simulink model "main"  (R2023b)
settings: Solver=VariableStepAuto  StartTime=0.0  StopTime=5  RelTol=1e-3
values from neighbouring files (symbols this model uses):
  IMU_sampling_rate = 0.02    [init.m]
  M_Bl = [ALTITUDE YAW -PITCH -ROLL]    [init.m]
  M_Br = [ALTITUDE -YAW -PITCH ROLL]    [init.m]
  M_fl = [ALTITUDE -YAW PITCH -ROLL]    [init.m]
  M_fr = [ALTITUDE YAW PITCH ROLL]    [init.m]
  Ts = 0.02    [init.m]
undefined symbols (not defined in the file or in its folder): dev, DiscIntNeverNeededParam, Main, pwm_output0
libraries: px4Sensorslib x6, slpidlib x4, cstblocks x4, simulink x4, px4lib x3, hdlsllib x2, etargetslib x2, mspfiltlib x1
settings Model: Creator=Jan  LastModifiedBy=Jan

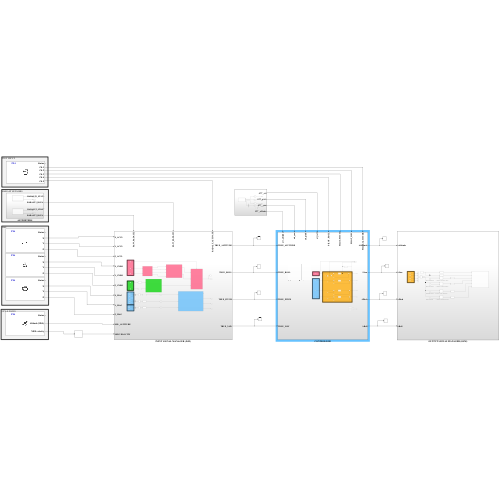
[thumbnail: Simulink's stored preview of the top-level diagram]
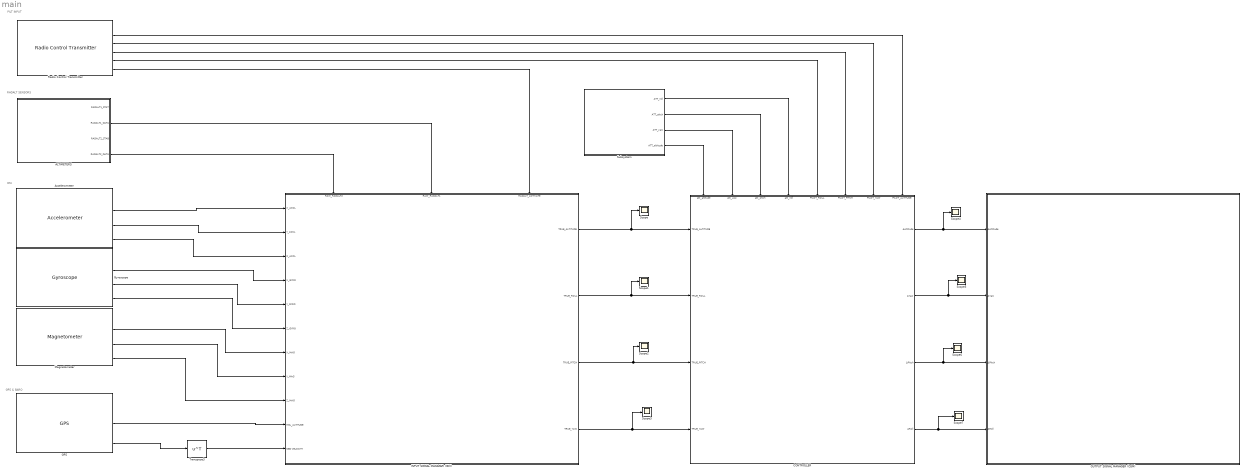
== system main ==
  note: IMU
  note: PILT INPUT
  note: RADALT SENSORS
  note: GPS & BARO
  ALTIMETERS : Subsystem
  Accelerometer : px4Sensorslib/Accelerometer  uorbTimeStamp=off  BlockingMode=off  BlockTimeout=1e-3  sampleTime=1/250
  CONTROLLER : Subsystem
      settings: PortSchema="{\"entries\":[{\"content\":{\"sides\":[{\"content\":{\"connectorIds\":[\"In1\",\"In2\",\"In3\",\"In4\"]},\"type\":\"ConnectorPlacement.EquallySpacedRectSide\",\"uuid\":\"b32f6c27-b4b4-43d4-a12f-bb52559986eb\"},{\"content\":{\"connectorIds\":[\"Out1\",\"Out2\",\"Out3\",\"Out4\"],\"side\":\"RIGHT\"},\"type\":\"ConnectorPlacement.EquallySpacedRectSide\",\"uuid\":\"bab16402-6e46-41ac-967f-b826d0c64ec3\"},{\"content\":{\"connectorIds\":[\"In5\",\"In6\",\"In7\",\"In8\",\"In9\",\"In10\",\"In11\",\"In12\"],\"side\":\"TOP\"},\"type\":\"ConnectorPlacement.EquallySpacedRectSide\",\"uuid\":\"8db3a1c8-77f2-471c-a34f-57b18e4d0f71\"},{\"content\":{\"side\":\"BOTTOM\"},\"type\":\"ConnectorPlacement.EquallySpacedRectSide\",\"uuid\":\"21d3ea43-ab92-4b57-8a2f-eb82c82d00b8\"}]},\"type\":\"ConnectorPlacement.EquallySpacedConnector\",\"uuid\":\"b37a3fa7-6be5-403c-bb68-9dda96af472d\"}],\"packageUris\":[\"http://schema.mathworks.com/mf0/Connector/R2020b\"],\"version\":\"1.0\"}"
  GPS : px4Sensorslib/GPS  lat=off  lon=off  alt=on  velocity=off  course=off  gpsfix=off  numsat=off  timestamp_utc=off  BlockingMode=off  BlockTimeout=1e-3  dop=off  vel_ned=on  alt_ellipsoid=off  jamm_ind=off  timestamp=off  sampleTime=1/250
  Gyroscope : px4Sensorslib/Gyroscope  uorbTimeStamp=off  BlockingMode=off  BlockTimeout=1e-3  sampleTime=1/250
  INPUT SIGNAL MANAGER (ISM) : Subsystem
      settings: PortSchema="{\"entries\":[{\"content\":{\"sides\":[{\"content\":{\"connectorIds\":[\"In1\",\"In2\",\"In3\",\"In4\",\"In5\",\"In6\",\"In7\",\"In8\",\"In9\",\"In10\",\"In11\"]},\"type\":\"ConnectorPlacement.EquallySpacedRectSide\",\"uuid\":\"5b240cc7-ef56-4424-b991-67f01d80d984\"},{\"content\":{\"connectorIds\":[\"Out1\",\"Out2\",\"Out3\",\"Out4\"],\"side\":\"RIGHT\"},\"type\":\"ConnectorPlacement.EquallySpacedRectSide\",\"uuid\":\"4a4e274e-121a-48d3-8cee-a4467ab5abd6\"},{\"content\":{\"connectorIds\":[\"In12\",\"In13\",\"In14\"],\"side\":\"TOP\"},\"type\":\"ConnectorPlacement.EquallySpacedRectSide\",\"uuid\":\"2d4a7b98-56a4-4ac1-89f6-3bfeef007e92\"}]},\"type\":\"ConnectorPlacement.EquallySpacedConnector\",\"uuid\":\"f5ce809e-f10f-4f9c-bc11-40e98aa3c504\"}],\"packageUris\":[\"http://schema.mathworks.com/mf0/Connector/R2020b\"],\"version\":\"1.0\"}"
  Magnetometer : px4Sensorslib/Magnetometer  uorbTimeStamp=off  BlockingMode=off  BlockTimeout=1e-3  sampleTime=1/250
  OUTPUT SIGNAL MANAGER (OSM) : Subsystem
  Radio Control Transmitter : px4Sensorslib/Radio Control Transmitter  channel1=on  channel2=on  channel3=on  channel4=on  channel5=on  channel6=off  channel7=off  channel8=off  channel_count=off  rssi=off  rc_input_source=off  timestamp_last_signal=off  time_stamp=off  sampleTime=1/250  BlockingMode=off  BlockTimeout=5
  Scope{,1..7} (8 alike) : Scope
  Subsystem : Subsystem
  Transpose3 : Math  Operator=transpose
  wires:
  ALTIMETERS/2(RADALT1_DATA) -> INPUT SIGNAL MANAGER (ISM)/13(RAW_RADALT1)
  ALTIMETERS/4(RADALT2_DATA) -> INPUT SIGNAL MANAGER (ISM)/12(RAW_RADALT2)
  Accelerometer/2 -> INPUT SIGNAL MANAGER (ISM)/1(X_ACCL)
  Accelerometer/3 -> INPUT SIGNAL MANAGER (ISM)/2(Y_ACCL)
  Accelerometer/4 -> INPUT SIGNAL MANAGER (ISM)/3(Z_ACCL)
  Gyroscope/2 -> INPUT SIGNAL MANAGER (ISM)/4(X_GYRO)
  Gyroscope/3 -> INPUT SIGNAL MANAGER (ISM)/5(Y_GYRO)
  Gyroscope/4 -> INPUT SIGNAL MANAGER (ISM)/6(Z_GYRO)
  Magnetometer/2 -> INPUT SIGNAL MANAGER (ISM)/7(X_MAG)
  Magnetometer/3 -> INPUT SIGNAL MANAGER (ISM)/8(Y_MAG)
  Magnetometer/4 -> INPUT SIGNAL MANAGER (ISM)/9(Z_MAG)
  GPS/3 -> Transpose3/1
  Transpose3/1 -> INPUT SIGNAL MANAGER (ISM)/11(NED VELOCITY)
  INPUT SIGNAL MANAGER (ISM)/2(TRUE_ROLL) -> Scope1/1, CONTROLLER/2(TRUE_ROLL)
  INPUT SIGNAL MANAGER (ISM)/4(TRUE_YAW) -> Scope3/1, CONTROLLER/4(TRUE_YAW)
  INPUT SIGNAL MANAGER (ISM)/3(TRUE_PITCH) -> Scope2/1, CONTROLLER/3(TRUE_PITCH)
  INPUT SIGNAL MANAGER (ISM)/1(TRUE_ALTITUDE) -> Scope/1, CONTROLLER/1(TRUE_ALTITUDE)
  Radio Control Transmitter/2 -> CONTROLLER/12(PILOT_ALTITUDE)
  Radio Control Transmitter/3 -> CONTROLLER/11(PILOT_YAW)
  Radio Control Transmitter/4 -> CONTROLLER/10(PILOT_PITCH)
  Radio Control Transmitter/5 -> CONTROLLER/9(PILOT_ROLL)
  CONTROLLER/1(ΔAltitude) -> Scope4/1, OUTPUT SIGNAL MANAGER (OSM)/1(ΔAltitude)
  CONTROLLER/2(ΔYaw) -> Scope5/1, OUTPUT SIGNAL MANAGER (OSM)/2(ΔYaw)
  CONTROLLER/3(ΔPitch) -> Scope6/1, OUTPUT SIGNAL MANAGER (OSM)/3(ΔPitch)
  CONTROLLER/4(ΔRoll) -> Scope7/1, OUTPUT SIGNAL MANAGER (OSM)/4(ΔRoll)
  Radio Control Transmitter/6 -> INPUT SIGNAL MANAGER (ISM)/14(RADALT_ACTIVATE)
  Subsystem/4(ATT_altitude) -> CONTROLLER/5(att_altitude)
  Subsystem/3(ATT_yaw) -> CONTROLLER/6(att_yaw)
  Subsystem/2(ATT_pitch) -> CONTROLLER/7(att_pitch)
  Subsystem/1(ATT_roll) -> CONTROLLER/8(att_roll)
  GPS/2 -> INPUT SIGNAL MANAGER (ISM)/10(MSL_ALTITUDE)

== system main/ALTIMETERS ==
  RADALT1 : px4lib/Serial Receive  SCIModule=/dev/ttyS6  DataType=uint8  DataLength=6  OutputStatus=on  SampleTime=1/2400  BlockingMode=off  PartialData=off  Timeout=5
  RADALT2 : px4lib/Serial Receive  SCIModule=/dev/ttyS3  DataType=uint8  DataLength=6  OutputStatus=on  SampleTime=1/2400  BlockingMode=off  PartialData=off  Timeout=5
  RADALT1_STAT : Outport
  RADALT1_DATA : Outport  Port=2
  RADALT2_STAB : Outport  Port=3
  RADALT2_DATA : Outport  Port=4
  wires:
  RADALT2/1 -> RADALT2_DATA/1  "RADALT2"
  RADALT1/1 -> RADALT1_DATA/1  "RADALT1"
  RADALT2/2 -> RADALT2_STAB/1
  RADALT1/2 -> RADALT1_STAT/1

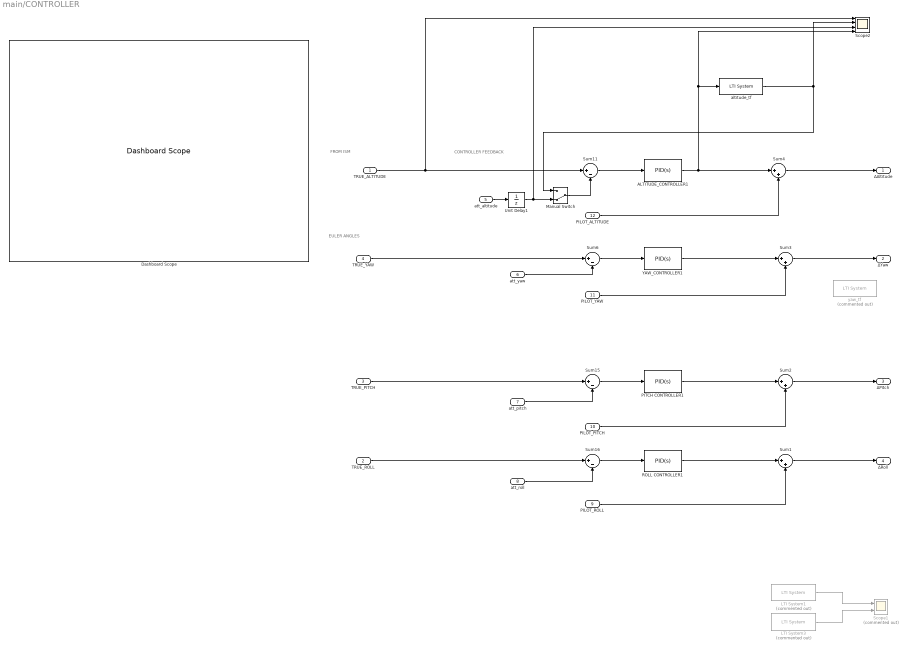
== system main/CONTROLLER ==
  note: EULER ANGLES
  note: FROM ISM
  note: CONTROLLER FEEDBACK
  TRUE_ALTITUDE : Inport
  TRUE_ROLL : Inport  Port=2
  TRUE_PITCH : Inport  Port=3
  TRUE_YAW : Inport  Port=4
  att_altitude : Inport  Port=5
  att_yaw : Inport  Port=6
  att_pitch : Inport  Port=7
  att_roll : Inport  Port=8
  PILOT_ROLL : Inport  Port=9
  PILOT_PITCH : Inport  Port=10
  PILOT_YAW : Inport  Port=11
  PILOT_ALTITUDE : Inport  Port=12
  ALTITUDE_CONTROLLER1 : slpidlib/PID Controller  Controller=PID  Form=Parallel  TimeDomain=Continuous-time  UseExternalTs=off  SampleTime=-1  IntegratorMethod=Forward Euler  FilterMethod=Forward Euler  ControllerParametersSource=internal  P=18932435531.83  I=88617163235.3465  UseKiTs=off  D=988633118.458494  N=575.969167967075  UseFilter=on  TunerSelectOption=Transfer Function Based (PID Tuner App)  InitialConditionSource=internal  InitialConditionForIntegrator=0  InitialConditionForFilter=0  DifferentiatorICPrevScaledInput=0  ExternalReset=none  TrackingMode=off  Kt=1  LimitOutput=off  SatLimitsSource=internal  UpperSaturationLimit=inf  LowerSaturationLimit=-inf  LinearizeAsGain=on  AntiWindupMode=none  Kb=1  LimitIntegrator=off  UpperIntegratorSaturationLimit=inf  LowerIntegratorSaturationLimit=-inf  POutMin=[]  POutMax=[]  IOutMin=[]  IOutMax=[]  DOutMin=[]  DOutMax=[]  NOutMin=[]  NOutMax=[]  SumOutMin=[]  SumOutMax=[]  SaturationOutMin=[]  SaturationOutMax=[]  PParamMin=[]  PParamMax=[]  IParamMin=[]  IParamMax=[]  DParamMin=[]  DParamMax=[]  NParamMin=[]  NParamMax=[]  KbParamMin=[]  KbParamMax=[]  KtParamMin=[]  KtParamMax=[]  KbOutMin=[]  KbOutMax=[]  KtOutMin=[]  KtOutMax=[]  IntegratorOutMin=[]  IntegratorOutMax=[]  FilterOutMin=[]  FilterOutMax=[]  SumI1OutMin=[]  SumI1OutMax=[]  SumI2OutMin=[]  SumI2OutMax=[]  SumI3OutMin=[]  SumI3OutMax=[]  SumI4OutMin=[]  SumI4OutMax=[]  SumDOutMin=[]  SumDOutMax=[]  DifferentiatorOutMin=[]  DifferentiatorOutMax=[]  FilterDiffOutCoefMin=[]  FilterDiffOutCoefMax=[]  ReciprocalOutMin=[]  ReciprocalOutMax=[]  SumDenOutMin=[]  SumDenOutMax=[]  SumNumOutMin=[]  SumNumOutMax=[]  DivideOutMin=[]  DivideOutMax=[]  UdiffTsProdOutMin=[]  UdiffTsProdOutMax=[]  NTsProdOutMin=[]  NTsProdOutMax=[]  UintegralTsProdOutMin=[]  UintegralTsProdOutMax=[]  UngainTsProdOutMin=[]  UngainTsProdOutMax=[]  ClampingZeroOutDataTypeStr=Inherit: Inherit via back propagation  ClampingZeroOutMin=[]  ClampingZeroOutMax=[]  FilterDenConstantOutDataTypeStr=Inherit: Inherit via back propagation  FilterDenConstantOutMin=[]  FilterDenConstantOutMax=[]  PCopyOutDataTypeStr=Inherit: Inherit via back propagation  PCopyOutMin=[]  PCopyOutMax=[]  NCopyOutDataTypeStr=Inherit: Inherit via back propagation  NCopyOutMin=[]  NCopyOutMax=[]  IntegratorContinuousStateAttributes=''  IntegratorStateMustResolveToSignalObject=off  IntegratorRTWStateStorageClass=Auto  FilterContinuousStateAttributes=''  FilterStateMustResolveToSignalObject=off  FilterRTWStateStorageClass=Auto  ParallelPVariant=InternalParameters  IdealPVariant=Disabled  IVariant=InternalParameters  DVariant=InternalParameters  IntegratorVariant=Continuous  SatVariant=Disabled  AWVariant=Passthrough  PCopyVariant=Disabled  TRVariant=Disabled  FdbkBlocksVariant=Forward  IdealPFdbkVariant=Disabled  SatFdbkVariant=Disabled  DerivativeFilterVariant=ContFilter  NVariant=InternalParameters  NCopyVariant=Disabled  FilterICVariant=InternalICsFilter  IntegratorICVariant=InternalICs  ExternalResetVariant=Disabled  TRSumVariant=Passthrough  SumFdbkVariant=Disabled  SumVariant=Sum_PID  TsampFilterVariant=InternalTs  TsampNgainVariant=Passthrough  TsampIntegralVariant=Disabled_SignalSpec  ExternalSaturationOutDataTypeStr=Inherit: Same as second input
  Dashboard Scope : DashboardScope  Ymin=-2  Ymax=10
  LTI System1 : cstblocks/LTI System  Commented=on  sys=pitch_tf  IC=[]  PadeOrder=0
  LTI System3 : cstblocks/LTI System  Commented=on  sys=roll_tf  IC=[]  PadeOrder=0
  Manual Switch : ManualSwitch  CurrentSetting=0
  PITCH CONTROLLER1 : slpidlib/PID Controller  Controller=PID  Form=Parallel  TimeDomain=Continuous-time  UseExternalTs=off  SampleTime=-1  IntegratorMethod=Forward Euler  FilterMethod=Forward Euler  ControllerParametersSource=internal  P=12359690.9371967  I=6312506.2640545  UseKiTs=off  D=5964351.03647163  N=104.897155810233  UseFilter=on  TunerSelectOption=Transfer Function Based (PID Tuner App)  InitialConditionSource=internal  InitialConditionForIntegrator=0  InitialConditionForFilter=0  DifferentiatorICPrevScaledInput=0  ExternalReset=none  TrackingMode=off  Kt=1  LimitOutput=off  SatLimitsSource=internal  UpperSaturationLimit=inf  LowerSaturationLimit=-inf  LinearizeAsGain=on  AntiWindupMode=none  Kb=1  LimitIntegrator=off  UpperIntegratorSaturationLimit=inf  LowerIntegratorSaturationLimit=-inf  POutMin=[]  POutMax=[]  IOutMin=[]  IOutMax=[]  DOutMin=[]  DOutMax=[]  NOutMin=[]  NOutMax=[]  SumOutMin=[]  SumOutMax=[]  SaturationOutMin=[]  SaturationOutMax=[]  PParamMin=[]  PParamMax=[]  IParamMin=[]  IParamMax=[]  DParamMin=[]  DParamMax=[]  NParamMin=[]  NParamMax=[]  KbParamMin=[]  KbParamMax=[]  KtParamMin=[]  KtParamMax=[]  KbOutMin=[]  KbOutMax=[]  KtOutMin=[]  KtOutMax=[]  IntegratorOutMin=[]  IntegratorOutMax=[]  FilterOutMin=[]  FilterOutMax=[]  SumI1OutMin=[]  SumI1OutMax=[]  SumI2OutMin=[]  SumI2OutMax=[]  SumI3OutMin=[]  SumI3OutMax=[]  SumI4OutMin=[]  SumI4OutMax=[]  SumDOutMin=[]  SumDOutMax=[]  DifferentiatorOutMin=[]  DifferentiatorOutMax=[]  FilterDiffOutCoefMin=[]  FilterDiffOutCoefMax=[]  ReciprocalOutMin=[]  ReciprocalOutMax=[]  SumDenOutMin=[]  SumDenOutMax=[]  SumNumOutMin=[]  SumNumOutMax=[]  DivideOutMin=[]  DivideOutMax=[]  UdiffTsProdOutMin=[]  UdiffTsProdOutMax=[]  NTsProdOutMin=[]  NTsProdOutMax=[]  UintegralTsProdOutMin=[]  UintegralTsProdOutMax=[]  UngainTsProdOutMin=[]  UngainTsProdOutMax=[]  ClampingZeroOutDataTypeStr=Inherit: Inherit via back propagation  ClampingZeroOutMin=[]  ClampingZeroOutMax=[]  FilterDenConstantOutDataTypeStr=Inherit: Inherit via back propagation  FilterDenConstantOutMin=[]  FilterDenConstantOutMax=[]  PCopyOutDataTypeStr=Inherit: Inherit via back propagation  PCopyOutMin=[]  PCopyOutMax=[]  NCopyOutDataTypeStr=Inherit: Inherit via back propagation  NCopyOutMin=[]  NCopyOutMax=[]  IntegratorContinuousStateAttributes=''  IntegratorStateMustResolveToSignalObject=off  IntegratorRTWStateStorageClass=Auto  FilterContinuousStateAttributes=''  FilterStateMustResolveToSignalObject=off  FilterRTWStateStorageClass=Auto  ParallelPVariant=InternalParameters  IdealPVariant=Disabled  IVariant=InternalParameters  DVariant=InternalParameters  IntegratorVariant=Continuous  SatVariant=Disabled  AWVariant=Passthrough  PCopyVariant=Disabled  TRVariant=Disabled  FdbkBlocksVariant=Forward  IdealPFdbkVariant=Disabled  SatFdbkVariant=Disabled  DerivativeFilterVariant=ContFilter  NVariant=InternalParameters  NCopyVariant=Disabled  FilterICVariant=InternalICsFilter  IntegratorICVariant=InternalICs  ExternalResetVariant=Disabled  TRSumVariant=Passthrough  SumFdbkVariant=Disabled  SumVariant=Sum_PID  TsampFilterVariant=InternalTs  TsampNgainVariant=Passthrough  TsampIntegralVariant=Disabled_SignalSpec  ExternalSaturationOutDataTypeStr=Inherit: Same as second input
  ROLL CONTROLLER1 : slpidlib/PID Controller  Controller=PID  Form=Parallel  TimeDomain=Continuous-time  UseExternalTs=off  SampleTime=-1  IntegratorMethod=Forward Euler  FilterMethod=Forward Euler  ControllerParametersSource=internal  P=15168306.557733  I=7671855.54074978  UseKiTs=off  D=5885982.08806878  N=104.897155810233  UseFilter=on  TunerSelectOption=Transfer Function Based (PID Tuner App)  InitialConditionSource=internal  InitialConditionForIntegrator=0  InitialConditionForFilter=0  DifferentiatorICPrevScaledInput=0  ExternalReset=none  TrackingMode=off  Kt=1  LimitOutput=off  SatLimitsSource=internal  UpperSaturationLimit=inf  LowerSaturationLimit=-inf  LinearizeAsGain=on  AntiWindupMode=none  Kb=1  LimitIntegrator=off  UpperIntegratorSaturationLimit=inf  LowerIntegratorSaturationLimit=-inf  POutMin=[]  POutMax=[]  IOutMin=[]  IOutMax=[]  DOutMin=[]  DOutMax=[]  NOutMin=[]  NOutMax=[]  SumOutMin=[]  SumOutMax=[]  SaturationOutMin=[]  SaturationOutMax=[]  PParamMin=[]  PParamMax=[]  IParamMin=[]  IParamMax=[]  DParamMin=[]  DParamMax=[]  NParamMin=[]  NParamMax=[]  KbParamMin=[]  KbParamMax=[]  KtParamMin=[]  KtParamMax=[]  KbOutMin=[]  KbOutMax=[]  KtOutMin=[]  KtOutMax=[]  IntegratorOutMin=[]  IntegratorOutMax=[]  FilterOutMin=[]  FilterOutMax=[]  SumI1OutMin=[]  SumI1OutMax=[]  SumI2OutMin=[]  SumI2OutMax=[]  SumI3OutMin=[]  SumI3OutMax=[]  SumI4OutMin=[]  SumI4OutMax=[]  SumDOutMin=[]  SumDOutMax=[]  DifferentiatorOutMin=[]  DifferentiatorOutMax=[]  FilterDiffOutCoefMin=[]  FilterDiffOutCoefMax=[]  ReciprocalOutMin=[]  ReciprocalOutMax=[]  SumDenOutMin=[]  SumDenOutMax=[]  SumNumOutMin=[]  SumNumOutMax=[]  DivideOutMin=[]  DivideOutMax=[]  UdiffTsProdOutMin=[]  UdiffTsProdOutMax=[]  NTsProdOutMin=[]  NTsProdOutMax=[]  UintegralTsProdOutMin=[]  UintegralTsProdOutMax=[]  UngainTsProdOutMin=[]  UngainTsProdOutMax=[]  ClampingZeroOutDataTypeStr=Inherit: Inherit via back propagation  ClampingZeroOutMin=[]  ClampingZeroOutMax=[]  FilterDenConstantOutDataTypeStr=Inherit: Inherit via back propagation  FilterDenConstantOutMin=[]  FilterDenConstantOutMax=[]  PCopyOutDataTypeStr=Inherit: Inherit via back propagation  PCopyOutMin=[]  PCopyOutMax=[]  NCopyOutDataTypeStr=Inherit: Inherit via back propagation  NCopyOutMin=[]  NCopyOutMax=[]  IntegratorContinuousStateAttributes=''  IntegratorStateMustResolveToSignalObject=off  IntegratorRTWStateStorageClass=Auto  FilterContinuousStateAttributes=''  FilterStateMustResolveToSignalObject=off  FilterRTWStateStorageClass=Auto  ParallelPVariant=InternalParameters  IdealPVariant=Disabled  IVariant=InternalParameters  DVariant=InternalParameters  IntegratorVariant=Continuous  SatVariant=Disabled  AWVariant=Passthrough  PCopyVariant=Disabled  TRVariant=Disabled  FdbkBlocksVariant=Forward  IdealPFdbkVariant=Disabled  SatFdbkVariant=Disabled  DerivativeFilterVariant=ContFilter  NVariant=InternalParameters  NCopyVariant=Disabled  FilterICVariant=InternalICsFilter  IntegratorICVariant=InternalICs  ExternalResetVariant=Disabled  TRSumVariant=Passthrough  SumFdbkVariant=Disabled  SumVariant=Sum_PID  TsampFilterVariant=InternalTs  TsampNgainVariant=Passthrough  TsampIntegralVariant=Disabled_SignalSpec  ExternalSaturationOutDataTypeStr=Inherit: Same as second input
  Scope1 : Scope  Commented=on  NumInputPorts=2
  Scope2 : Scope  NumInputPorts=4
  Sum{1..4} (4 alike) : Sum  Inputs=|++
  Sum{6,11,15..16} (4 alike) : Sum  Inputs=|+-
  Unit Delay1 : UnitDelay  SampleTime=-1  HasFrameUpgradeWarning=on
  YAW_CONTROLLER1 : slpidlib/PID Controller  Controller=PID  Form=Parallel  TimeDomain=Continuous-time  UseExternalTs=off  SampleTime=-1  IntegratorMethod=Forward Euler  FilterMethod=Forward Euler  ControllerParametersSource=internal  P=834762470.893906  I=422207783.259263  UseKiTs=off  D=323925214.246719  N=104.897155810233  UseFilter=on  TunerSelectOption=Transfer Function Based (PID Tuner App)  InitialConditionSource=internal  InitialConditionForIntegrator=0  InitialConditionForFilter=0  DifferentiatorICPrevScaledInput=0  ExternalReset=none  TrackingMode=off  Kt=1  LimitOutput=off  SatLimitsSource=internal  UpperSaturationLimit=inf  LowerSaturationLimit=-inf  LinearizeAsGain=on  AntiWindupMode=none  Kb=1  LimitIntegrator=off  UpperIntegratorSaturationLimit=inf  LowerIntegratorSaturationLimit=-inf  POutMin=[]  POutMax=[]  IOutMin=[]  IOutMax=[]  DOutMin=[]  DOutMax=[]  NOutMin=[]  NOutMax=[]  SumOutMin=[]  SumOutMax=[]  SaturationOutMin=[]  SaturationOutMax=[]  PParamMin=[]  PParamMax=[]  IParamMin=[]  IParamMax=[]  DParamMin=[]  DParamMax=[]  NParamMin=[]  NParamMax=[]  KbParamMin=[]  KbParamMax=[]  KtParamMin=[]  KtParamMax=[]  KbOutMin=[]  KbOutMax=[]  KtOutMin=[]  KtOutMax=[]  IntegratorOutMin=[]  IntegratorOutMax=[]  FilterOutMin=[]  FilterOutMax=[]  SumI1OutMin=[]  SumI1OutMax=[]  SumI2OutMin=[]  SumI2OutMax=[]  SumI3OutMin=[]  SumI3OutMax=[]  SumI4OutMin=[]  SumI4OutMax=[]  SumDOutMin=[]  SumDOutMax=[]  DifferentiatorOutMin=[]  DifferentiatorOutMax=[]  FilterDiffOutCoefMin=[]  FilterDiffOutCoefMax=[]  ReciprocalOutMin=[]  ReciprocalOutMax=[]  SumDenOutMin=[]  SumDenOutMax=[]  SumNumOutMin=[]  SumNumOutMax=[]  DivideOutMin=[]  DivideOutMax=[]  UdiffTsProdOutMin=[]  UdiffTsProdOutMax=[]  NTsProdOutMin=[]  NTsProdOutMax=[]  UintegralTsProdOutMin=[]  UintegralTsProdOutMax=[]  UngainTsProdOutMin=[]  UngainTsProdOutMax=[]  ClampingZeroOutDataTypeStr=Inherit: Inherit via back propagation  ClampingZeroOutMin=[]  ClampingZeroOutMax=[]  FilterDenConstantOutDataTypeStr=Inherit: Inherit via back propagation  FilterDenConstantOutMin=[]  FilterDenConstantOutMax=[]  PCopyOutDataTypeStr=Inherit: Inherit via back propagation  PCopyOutMin=[]  PCopyOutMax=[]  NCopyOutDataTypeStr=Inherit: Inherit via back propagation  NCopyOutMin=[]  NCopyOutMax=[]  IntegratorContinuousStateAttributes=''  IntegratorStateMustResolveToSignalObject=off  IntegratorRTWStateStorageClass=Auto  FilterContinuousStateAttributes=''  FilterStateMustResolveToSignalObject=off  FilterRTWStateStorageClass=Auto  ParallelPVariant=InternalParameters  IdealPVariant=Disabled  IVariant=InternalParameters  DVariant=InternalParameters  IntegratorVariant=Continuous  SatVariant=Disabled  AWVariant=Passthrough  PCopyVariant=Disabled  TRVariant=Disabled  FdbkBlocksVariant=Forward  IdealPFdbkVariant=Disabled  SatFdbkVariant=Disabled  DerivativeFilterVariant=ContFilter  NVariant=InternalParameters  NCopyVariant=Disabled  FilterICVariant=InternalICsFilter  IntegratorICVariant=InternalICs  ExternalResetVariant=Disabled  TRSumVariant=Passthrough  SumFdbkVariant=Disabled  SumVariant=Sum_PID  TsampFilterVariant=InternalTs  TsampNgainVariant=Passthrough  TsampIntegralVariant=Disabled_SignalSpec  ExternalSaturationOutDataTypeStr=Inherit: Same as second input
  altitude_tf : cstblocks/LTI System  sys=altitude_tf  IC=[]  PadeOrder=0
  yaw_tf : cstblocks/LTI System  Commented=on  sys=yaw_tf  IC=[]  PadeOrder=0
  ΔAltitude : Outport
  ΔYaw : Outport  Port=2
  ΔPitch : Outport  Port=3
  ΔRoll : Outport  Port=4
  wires:
  YAW_CONTROLLER1/1 -> Sum3/1
  Sum4/1 -> ΔAltitude/1
  ROLL CONTROLLER1/1 -> Sum1/1
  PILOT_ALTITUDE/1 -> Sum4/2
  PILOT_YAW/1 -> Sum3/2
  Sum16/1 -> ROLL CONTROLLER1/1
  Sum1/1 -> ΔRoll/1
  PILOT_ROLL/1 -> Sum1/2
  PITCH CONTROLLER1/1 -> Sum2/1
  Sum15/1 -> PITCH CONTROLLER1/1
  ALTITUDE_CONTROLLER1/1 -> Scope2/4, altitude_tf/1, Sum4/1
  Sum2/1 -> ΔPitch/1
  PILOT_PITCH/1 -> Sum2/2
  Sum11/1 -> ALTITUDE_CONTROLLER1/1
  Sum6/1 -> YAW_CONTROLLER1/1
  TRUE_ROLL/1 -> Sum16/1
  TRUE_PITCH/1 -> Sum15/1
  TRUE_YAW/1 -> Sum6/1
  TRUE_ALTITUDE/1 -> Scope2/1, Sum11/1
  att_yaw/1 -> Sum6/2
  att_pitch/1 -> Sum15/2
  att_roll/1 -> Sum16/2
  Sum3/1 -> ΔYaw/1
  LTI System1/1 -> Scope1/1
  LTI System3/1 -> Scope1/2
  Manual Switch/1 -> Sum11/2
  altitude_tf/1 -> Manual Switch/1, Scope2/2
  Unit Delay1/1 -> Scope2/3, Manual Switch/2
  att_altitude/1 -> Unit Delay1/1

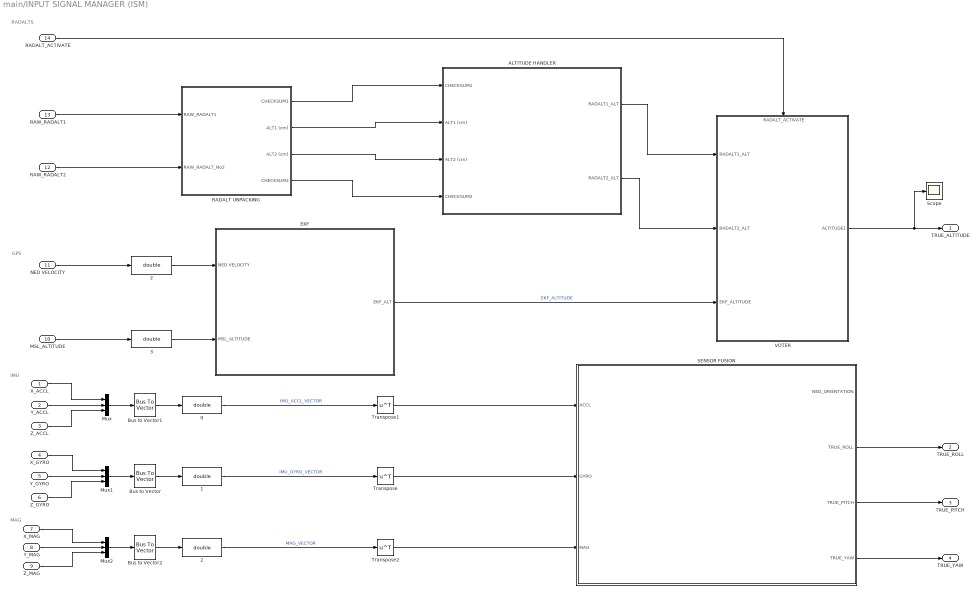
== system main/INPUT SIGNAL MANAGER (ISM) ==
  note: GPS
  note: RADALTS
  note: IMU
  note: MAG
  X_ACCL : Inport
  Y_ACCL : Inport  Port=2
  Z_ACCL : Inport  Port=3
  X_GYRO : Inport  Port=4
  Y_GYRO : Inport  Port=5
  Z_GYRO : Inport  Port=6
  X_MAG : Inport  Port=7
  Y_MAG : Inport  Port=8
  Z_MAG : Inport  Port=9
  MSL_ALTITUDE : Inport  Port=10
  NED VELOCITY : Inport  Port=11
  RAW_RADALT2 : Inport  Port=12
  RAW_RADALT1 : Inport  Port=13
  RADALT_ACTIVATE : Inport  Port=14
  " 2" : DataTypeConversion  OutDataTypeStr=double  SaturateOnIntegerOverflow=off  RndMeth=Floor
  "0 " : DataTypeConversion  OutDataTypeStr=double  SaturateOnIntegerOverflow=off  RndMeth=Floor
  1 : DataTypeConversion  OutDataTypeStr=double  SaturateOnIntegerOverflow=off  RndMeth=Floor
  2 : DataTypeConversion  OutDataTypeStr=double  SaturateOnIntegerOverflow=off  RndMeth=Floor
  3 : DataTypeConversion  OutDataTypeStr=double  SaturateOnIntegerOverflow=off  RndMeth=Floor
  ALTITUDE HANDLER : Subsystem
  Bus to Vector : BusToVector
  Bus to Vector1 : BusToVector
  Bus to Vector2 : BusToVector
  EKF : Subsystem
  Mux : Mux  Inputs=3
  Mux1 : Mux  Inputs=3
  Mux2 : Mux  Inputs=3
  RADALT UNPACKING : Subsystem
  SENSOR FUSION : Subsystem
  Scope : Scope
  Transpose : Math  Operator=transpose
  Transpose1 : Math  Operator=transpose
  Transpose2 : Math  Operator=transpose
  VOTER : Subsystem
      settings: PortSchema="{\"entries\":[{\"content\":{\"sides\":[{\"content\":{\"connectorIds\":[\"In1\",\"In2\",\"In3\"]},\"type\":\"ConnectorPlacement.EquallySpacedRectSide\",\"uuid\":\"dc1c39ce-0403-459b-94e1-ddedc0ea1ee4\"},{\"content\":{\"connectorIds\":[\"Out1\"],\"side\":\"RIGHT\"},\"type\":\"ConnectorPlacement.EquallySpacedRectSide\",\"uuid\":\"853442a8-64b8-4778-9114-161db545e8e2\"},{\"content\":{\"connectorIds\":[\"In4\"],\"side\":\"TOP\"},\"type\":\"ConnectorPlacement.EquallySpacedRectSide\",\"uuid\":\"2ebd7c90-ed78-4be6-83fb-fb9bd20822eb\"}]},\"type\":\"ConnectorPlacement.EquallySpacedConnector\",\"uuid\":\"d02cc3c8-2437-46b2-8909-af6c76dce3d6\"}],\"packageUris\":[\"http://schema.mathworks.com/mf0/Connector/R2020b\"],\"version\":\"1.0\"}"
  TRUE_ALTITUDE : Outport
  TRUE_ROLL : Outport  Port=2
  TRUE_PITCH : Outport  Port=3
  TRUE_YAW : Outport  Port=4
  wires:
  RAW_RADALT1/1 -> RADALT UNPACKING/1(RAW_RADALT1)
  RAW_RADALT2/1 -> RADALT UNPACKING/2(RAW_RADALT_No2)
  RADALT UNPACKING/2(ALT1 (cm)) -> ALTITUDE HANDLER/2(ALT1 (cm))
  RADALT UNPACKING/3(ALT2 (cm)) -> ALTITUDE HANDLER/3(ALT2 (cm))
  RADALT UNPACKING/1(CHECKSUM1) -> ALTITUDE HANDLER/1(CHECKSUM1)
  RADALT UNPACKING/4(CHECKSUM2) -> ALTITUDE HANDLER/4(CHECKSUM2)
  X_ACCL/1 -> Mux/1
  Y_ACCL/1 -> Mux/2
  Z_ACCL/1 -> Mux/3
  X_GYRO/1 -> Mux1/1
  Y_GYRO/1 -> Mux1/2
  Z_GYRO/1 -> Mux1/3
  Mux/1 -> Bus to Vector1/1
  Mux1/1 -> Bus to Vector/1
  Mux2/1 -> Bus to Vector2/1
  Y_MAG/1 -> Mux2/2
  Z_MAG/1 -> Mux2/3
  X_MAG/1 -> Mux2/1
  " 2"/1 -> Transpose2/1  "MAG_VECTOR"
  "0 "/1 -> Transpose1/1  "IMU_ACCL_VECTOR"
  1/1 -> Transpose/1  "IMU_GYRO_VECTOR"
  NED VELOCITY/1 -> 2/1
  Transpose/1 -> SENSOR FUSION/2(GYRO)
  Transpose1/1 -> SENSOR FUSION/1(ACCL)
  Transpose2/1 -> SENSOR FUSION/3(MAG)
  SENSOR FUSION/3(TRUE_PITCH) -> TRUE_PITCH/1
  SENSOR FUSION/2(TRUE_ROLL) -> TRUE_ROLL/1
  SENSOR FUSION/4(TRUE_YAW) -> TRUE_YAW/1
  ALTITUDE HANDLER/1(RADALT1_ALT) -> VOTER/1(RADALT1_ALT)
  ALTITUDE HANDLER/2(RADALT2_ALT) -> VOTER/2(RADALT2_ALT)
  VOTER/1(ALTITUDE1) -> Scope/1, TRUE_ALTITUDE/1
  Bus to Vector2/1 -> " 2"/1
  Bus to Vector/1 -> 1/1
  Bus to Vector1/1 -> "0 "/1
  MSL_ALTITUDE/1 -> 3/1
  RADALT_ACTIVATE/1 -> VOTER/4(RADALT_ACTIVATE)
  EKF/1(EKF_ALT) -> VOTER/3(EKF_ALTITUDE)  "EKF_ALTITUDE"
  2/1 -> EKF/1(NED VELOCITY)
  3/1 -> EKF/2(MSL_ALTITUDE)

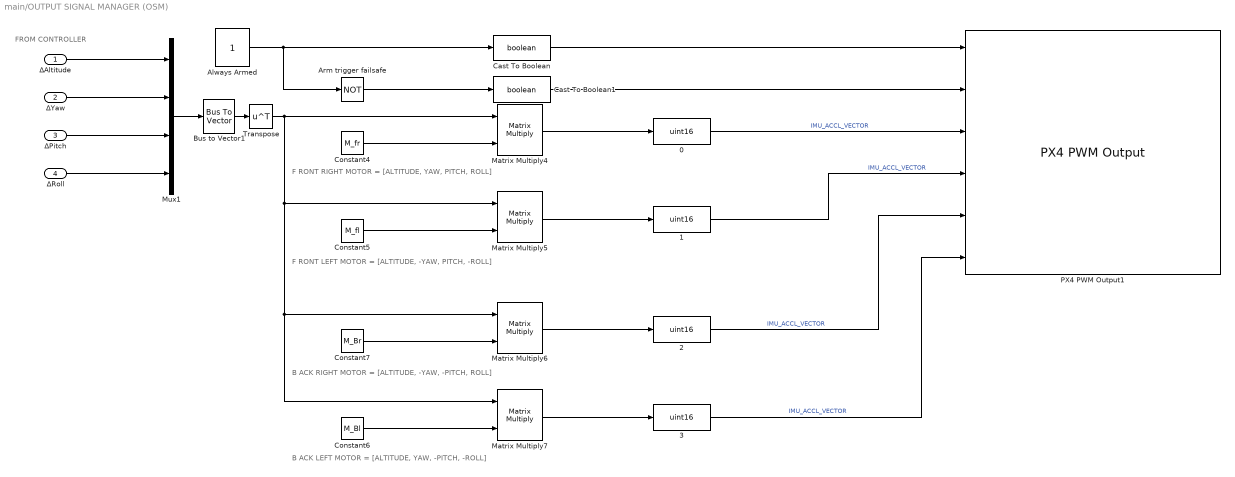
== system main/OUTPUT SIGNAL MANAGER (OSM) ==
  note: FROM CONTROLLER
  note: B ACK LEFT MOTOR = [ALTITUDE, YAW, -PITCH, -ROLL]
  note: F RONT LEFT MOTOR = [ALTITUDE, -YAW, PITCH, -ROLL]
  note: B ACK RIGHT MOTOR = [ALTITUDE, -YAW, -PITCH, ROLL]
  note: F RONT RIGHT MOTOR = [ALTITUDE, YAW, PITCH, ROLL]
  ΔAltitude : Inport
  ΔYaw : Inport  Port=2
  ΔPitch : Inport  Port=3
  ΔRoll : Inport  Port=4
  {0..3} (4 alike) : DataTypeConversion  OutDataTypeStr=uint16  SaturateOnIntegerOverflow=off  RndMeth=Floor
  Always Armed : Constant
  Arm trigger failsafe : Logic  Operator=NOT  IconShape=distinctive  AllPortsSameDT=off  OutDataTypeStr=boolean
  Bus to Vector1 : BusToVector
  Cast To Boolean : DataTypeConversion  OutDataTypeStr=boolean  SaturateOnIntegerOverflow=off  RndMeth=Floor
  Cast To Boolean1 : DataTypeConversion  OutDataTypeStr=boolean  SaturateOnIntegerOverflow=off  RndMeth=Floor
  Constant4 : Constant  Value=M_fr
  Constant5 : Constant  Value=M_fl
  Constant6 : Constant  Value=M_Bl
  Constant7 : Constant  Value=M_Br
  Matrix Multiply{4..7} (4 alike) : Product  Multiplication=Matrix(*)
  Mux1 : Mux
  PX4 PWM Output1 : px4lib/PX4 PWM Output  pwmDevice=Main (/dev/pwm_output0)  pwmChannel1_=on  pwmChannel2_=on  pwmChannel3_=on  pwmChannel4_=on  pwmChannel5_=off  pwmChannel6_=off  pwmChannel7_=off  pwmChannel8_=off  forceTerminateFailsafe=off  outputErrorStatus=off
  Transpose : Math  Operator=transpose
  wires:
  Constant6/1 -> Matrix Multiply7/2
  ΔRoll/1 -> Mux1/4
  ΔAltitude/1 -> Mux1/1
  ΔYaw/1 -> Mux1/2
  ΔPitch/1 -> Mux1/3
  Mux1/1 -> Bus to Vector1/1
  Bus to Vector1/1 -> Transpose/1
  Constant4/1 -> Matrix Multiply4/2
  Constant7/1 -> Matrix Multiply6/2
  Always Armed/1 -> Cast To Boolean/1, Arm trigger failsafe/1
  Constant5/1 -> Matrix Multiply5/2
  Arm trigger failsafe/1 -> Cast To Boolean1/1
  Matrix Multiply5/1 -> 1/1
  1/1 -> PX4 PWM Output1/4  "IMU_ACCL_VECTOR"
  Matrix Multiply4/1 -> 0/1
  0/1 -> PX4 PWM Output1/3  "IMU_ACCL_VECTOR"
  Matrix Multiply6/1 -> 2/1
  2/1 -> PX4 PWM Output1/5  "IMU_ACCL_VECTOR"
  Matrix Multiply7/1 -> 3/1
  3/1 -> PX4 PWM Output1/6  "IMU_ACCL_VECTOR"
  Transpose/1 -> Matrix Multiply5/1, Matrix Multiply7/1, Matrix Multiply6/1, Matrix Multiply4/1
  Cast To Boolean/1 -> PX4 PWM Output1/1
  Cast To Boolean1/1 -> PX4 PWM Output1/2

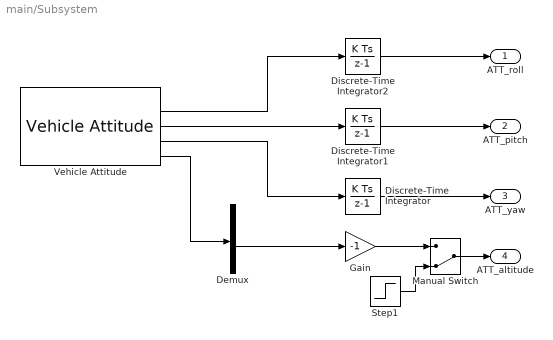
== system main/Subsystem ==
  Demux : Demux
  Discrete-Time Integrator : DiscreteIntegrator  SampleTime=-1  ICPrevOutput=DiscIntNeverNeededParam  ICPrevScaledInput=DiscIntNeverNeededParam
  Discrete-Time Integrator1 : DiscreteIntegrator  SampleTime=-1  ICPrevOutput=DiscIntNeverNeededParam  ICPrevScaledInput=DiscIntNeverNeededParam
  Discrete-Time Integrator2 : DiscreteIntegrator  SampleTime=-1  ICPrevOutput=DiscIntNeverNeededParam  ICPrevScaledInput=DiscIntNeverNeededParam
  Gain : Gain  Gain=-1
  Manual Switch : ManualSwitch  CurrentSetting=0
  Step1 : Step  Time=10  Before=5  After=5  SampleTime=10
  Vehicle Attitude : px4Sensorslib/Vehicle Attitude  rollRate=on  pitchRate=on  yawRate=on  quaternion=on  uorbTimeStamp=off  BlockingMode=off  BlockTimeout=0.001  sampleTime=1/250
  ATT_roll : Outport
  ATT_pitch : Outport  Port=2
  ATT_yaw : Outport  Port=3
  ATT_altitude : Outport  Port=4
  wires:
  Vehicle Attitude/5 -> Demux/1
  Demux/3 -> Gain/1
  Vehicle Attitude/4 -> Discrete-Time Integrator/1
  Vehicle Attitude/3 -> Discrete-Time Integrator1/1
  Vehicle Attitude/2 -> Discrete-Time Integrator2/1
  Discrete-Time Integrator2/1 -> ATT_roll/1
  Discrete-Time Integrator1/1 -> ATT_pitch/1
  Discrete-Time Integrator/1 -> ATT_yaw/1
  Gain/1 -> Manual Switch/1
  Step1/1 -> Manual Switch/2
  Manual Switch/1 -> ATT_altitude/1

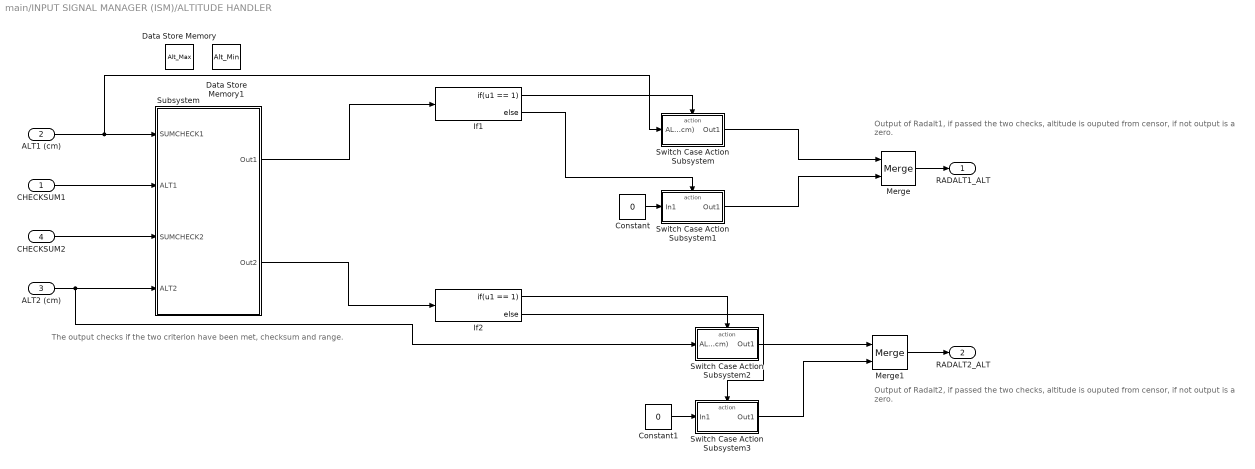
== system main/INPUT SIGNAL MANAGER (ISM)/ALTITUDE HANDLER ==
  note: The output checks if the two criterion have been met, checksum and range.
  note: Output of Radalt2, if passed the two checks, altitude is ouputed from censor, if not output is a zero.
  note: Output of Radalt1, if passed the two checks, altitude is ouputed from censor, if not output is a zero.
  CHECKSUM1 : Inport
  ALT1 (cm) : Inport  Port=2
  ALT2 (cm) : Inport  Port=3
  CHECKSUM2 : Inport  Port=4
  Constant : Constant  Value=0
  Constant1 : Constant  Value=0
  Data Store Memory : DataStoreMemory  DataStoreName=Alt_Max  WriteAfterWriteMsg=warning  ShowAdditionalParam=off
  Data Store Memory1 : DataStoreMemory  DataStoreName=Alt_Min  WriteAfterWriteMsg=warning  ShowAdditionalParam=off
  If1 : If  IfExpression=u1 == 1
  If2 : If  IfExpression=u1 == 1
  Merge : Merge
  Merge1 : Merge
  Subsystem : Subsystem
  Switch Case Action Subsystem : Subsystem  TreatAsAtomicUnit=on
  Switch Case Action Subsystem1 : Subsystem  TreatAsAtomicUnit=on
  Switch Case Action Subsystem2 : Subsystem  TreatAsAtomicUnit=on
  Switch Case Action Subsystem3 : Subsystem  TreatAsAtomicUnit=on
  RADALT1_ALT : Outport
  RADALT2_ALT : Outport  Port=2
  wires:
  Switch Case Action Subsystem3/1(Out1) -> Merge1/2
  Merge/1 -> RADALT1_ALT/1
  Merge1/1 -> RADALT2_ALT/1
  CHECKSUM1/1 -> Subsystem/2(ALT1)
  Switch Case Action Subsystem1/1(Out1) -> Merge/2
  If2/2 -> Switch Case Action Subsystem3/Action
  CHECKSUM2/1 -> Subsystem/3(SUMCHECK2)
  ALT2 (cm)/1 -> Switch Case Action Subsystem2/1(ALT2 (cm)), Subsystem/4(ALT2)
  If1/1 -> Switch Case Action Subsystem/Action
  Switch Case Action Subsystem2/1(Out1) -> Merge1/1
  If1/2 -> Switch Case Action Subsystem1/Action
  Subsystem/1(Out1) -> If1/1
  If2/1 -> Switch Case Action Subsystem2/Action
  Constant/1 -> Switch Case Action Subsystem1/1(In1)
  ALT1 (cm)/1 -> Switch Case Action Subsystem/1(ALT1 (cm)), Subsystem/1(SUMCHECK1)
  Constant1/1 -> Switch Case Action Subsystem3/1(In1)
  Switch Case Action Subsystem/1(Out1) -> Merge/1
  Subsystem/2(Out2) -> If2/1

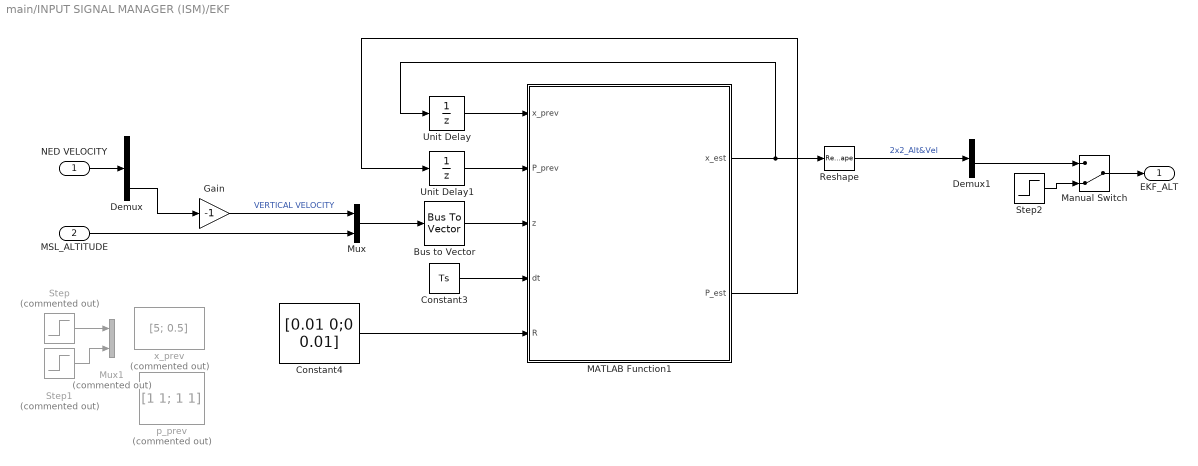
== system main/INPUT SIGNAL MANAGER (ISM)/EKF ==
  NED VELOCITY : Inport
  MSL_ALTITUDE : Inport  Port=2
  Bus to Vector : BusToVector
  Constant3 : Constant  Value=Ts
  Constant4 : Constant  Value=[0.01 0;0 0.01]
  Demux : Demux  Outputs=3
  Demux1 : Demux
  Gain : Gain  Gain=-1
  MATLAB Function1 : MATLAB Function  TreatAsAtomicUnit=on
  Manual Switch : ManualSwitch  CurrentSetting=0
  Mux : Mux  Inputs=2
  Mux1 : Mux  Commented=on  Inputs=2
  Reshape : Reshape
  Step : Step  Commented=on  Time=5  Before=5  After=5  SampleTime=0.02
  Step1 : Step  Commented=on  Time=5  Before=0.5  After=0.5  SampleTime=0.02
  Step2 : Step  Time=10  Before=5  After=5  SampleTime=1
  Unit Delay : UnitDelay  SampleTime=-1  HasFrameUpgradeWarning=on
  Unit Delay1 : UnitDelay  SampleTime=-1  HasFrameUpgradeWarning=on
  p_prev : Constant  Commented=on  Value=[1 1; 1 1]
  x_prev : Constant  Commented=on  Value=[5; 0.5]
  EKF_ALT : Outport
  wires:
  MSL_ALTITUDE/1 -> Mux/2
  Mux/1 -> Bus to Vector/1
  MATLAB Function1/2(P_est) -> Unit Delay1/1
  Constant4/1 -> MATLAB Function1/5(R)
  MATLAB Function1/1(x_est) -> Reshape/1, Unit Delay/1
  Unit Delay/1 -> MATLAB Function1/1(x_prev)
  Bus to Vector/1 -> MATLAB Function1/3(z)
  Constant3/1 -> MATLAB Function1/4(dt)
  Unit Delay1/1 -> MATLAB Function1/2(P_prev)
  Step1/1 -> Mux1/2
  Step/1 -> Mux1/1
  NED VELOCITY/1 -> Demux/1
  Demux/3 -> Gain/1
  Gain/1 -> Mux/1  "VERTICAL VELOCITY"
  Reshape/1 -> Demux1/1  "2x2_Alt&Vel"
  Step2/1 -> Manual Switch/2
  Demux1/3 -> Manual Switch/1
  Manual Switch/1 -> EKF_ALT/1

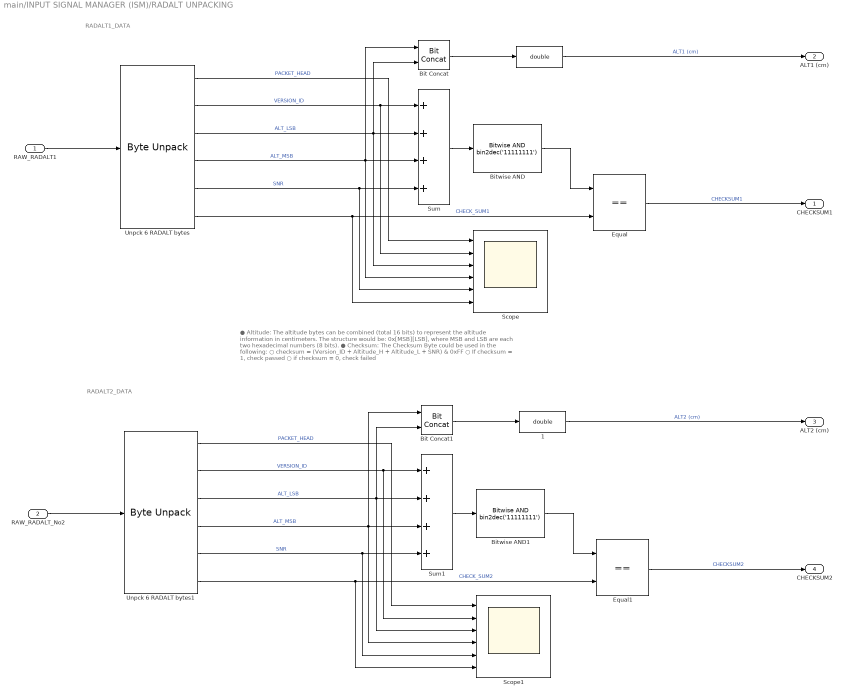
== system main/INPUT SIGNAL MANAGER (ISM)/RADALT UNPACKING ==
  note: RADALT2_DATA
  note: RADALT1_DATA
  note: ● Altitude: The altitude bytes can be combined (total 16 bits) to represent the altitude information in centimeters. The structure would be: 0x[MSB][LSB], where MSB and LSB are each two hexadecimal numbers (8 bits).
      | ● Checksum: The Checksum Byte could be used in the following:
      | ○ checksum = (Version_ID + Altitude_H + Altitude_L + SNR) & 0xFF
      | ○ If checksum = 1, check passed ○ if checksum = 0, check failed
  RAW_RADALT1 : Inport
  RAW_RADALT_No2 : Inport  Port=2
  " " : DataTypeConversion  OutDataTypeStr=double  SaturateOnIntegerOverflow=off  RndMeth=Floor
  " 1" : DataTypeConversion  OutDataTypeStr=double  SaturateOnIntegerOverflow=off  RndMeth=Floor
  Bit Concat : hdlsllib/Logic and Bit Operations/Bit Concat  numInputs=2
  Bit Concat1 : hdlsllib/Logic and Bit Operations/Bit Concat  numInputs=2
  Bitwise AND : simulink/Logic and Bit Operations/Bitwise Operator  logicop=AND  UseBitMask=on  BitMask=bin2dec('11111111')  BitMaskRealWorld=Stored Integer
      settings: LibrarySourceBlock=|
      | simulink/Quick Insert/Logic and Bit
      | Operations/Bitwise AND
  Bitwise AND1 : simulink/Logic and Bit Operations/Bitwise Operator  logicop=AND  UseBitMask=on  BitMask=bin2dec('11111111')  BitMaskRealWorld=Stored Integer
      settings: LibrarySourceBlock=|
      | simulink/Quick Insert/Logic and Bit
      | Operations/Bitwise AND
  Equal : RelationalOperator  Operator===  OutDataTypeStr=boolean  RndMeth=Simplest  InputSameDT=off
  Equal1 : RelationalOperator  Operator===  OutDataTypeStr=boolean  RndMeth=Simplest  InputSameDT=off
  Scope : Scope  NumInputPorts=6
  Scope1 : Scope  NumInputPorts=6
  Sum : Sum  Inputs=++++
  Sum1 : Sum  Inputs=++++
  Unpck 6 RADALT bytes : etargetslib/Byte Unpack  dimensions={[1],[1],[1],[1],[1],[1]}  datatypes={'uint8', 'uint8', 'uint8', 'uint8', 'uint8', 'uint8'}  byteAlign=1
      settings: LibrarySourceBlock=embeddedtargetslib/Host Communication/Byte Unpack
  Unpck 6 RADALT bytes1 : etargetslib/Byte Unpack  dimensions={[1],[1],[1],[1],[1],[1]}  datatypes={'uint8', 'uint8', 'uint8', 'uint8', 'uint8', 'uint8'}  byteAlign=1
      settings: LibrarySourceBlock=embeddedtargetslib/Host Communication/Byte Unpack
  CHECKSUM1 : Outport
  ALT1 (cm) : Outport  Port=2
  ALT2 (cm) : Outport  Port=3
  CHECKSUM2 : Outport  Port=4
  wires:
  Equal/1 -> CHECKSUM1/1  "CHECKSUM1"
  " "/1 -> ALT1 (cm)/1  "ALT1 (cm)"
  " 1"/1 -> ALT2 (cm)/1  "ALT2 (cm)"
  Equal1/1 -> CHECKSUM2/1  "CHECKSUM2"
  RAW_RADALT1/1 -> Unpck 6 RADALT bytes/1
  Bit Concat/1 -> " "/1
  Bitwise AND/1 -> Equal/1
  Unpck 6 RADALT bytes/6 -> Scope/6, Equal/2  "CHECK_SUM1"
  Unpck 6 RADALT bytes/3 -> Bit Concat/2, Scope/3, Sum/2  "ALT_LSB"
  Unpck 6 RADALT bytes/1 -> Scope/1  "PACKET_HEAD"
  Unpck 6 RADALT bytes/2 -> Scope/2, Sum/1  "VERSION_ID"
  Unpck 6 RADALT bytes/4 -> Bit Concat/1, Scope/4, Sum/3  "ALT_MSB"
  Sum/1 -> Bitwise AND/1
  Unpck 6 RADALT bytes/5 -> Scope/5, Sum/4  "SNR"
  RAW_RADALT_No2/1 -> Unpck 6 RADALT bytes1/1
  Bit Concat1/1 -> " 1"/1
  Unpck 6 RADALT bytes1/3 -> Bit Concat1/2, Scope1/3, Sum1/2  "ALT_LSB"
  Unpck 6 RADALT bytes1/2 -> Scope1/2, Sum1/1  "VERSION_ID"
  Unpck 6 RADALT bytes1/6 -> Scope1/6, Equal1/2  "CHECK_SUM2"
  Unpck 6 RADALT bytes1/5 -> Scope1/5, Sum1/4  "SNR"
  Bitwise AND1/1 -> Equal1/1
  Unpck 6 RADALT bytes1/4 -> Bit Concat1/1, Scope1/4, Sum1/3  "ALT_MSB"
  Unpck 6 RADALT bytes1/1 -> Scope1/1  "PACKET_HEAD"
  Sum1/1 -> Bitwise AND1/1

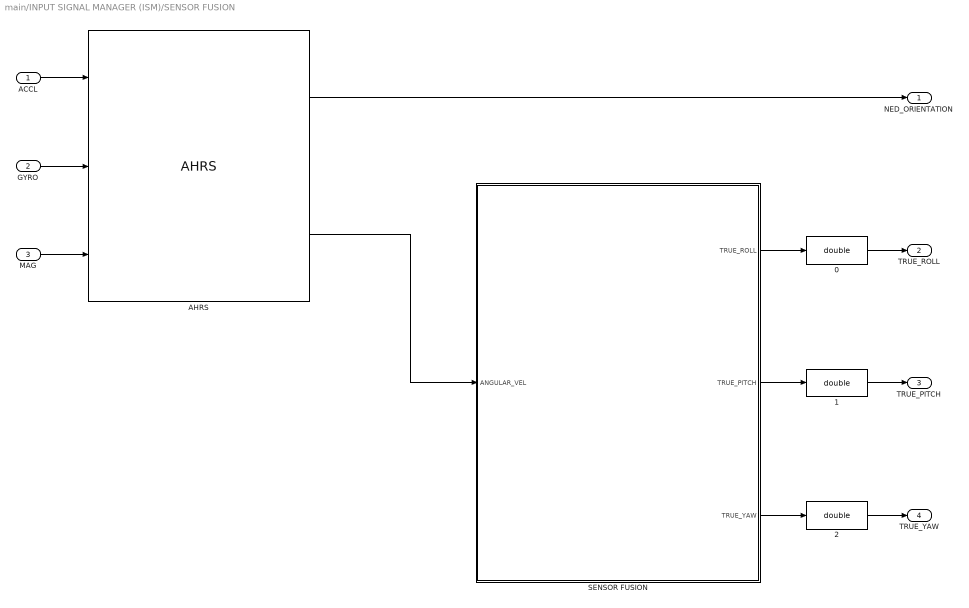
== system main/INPUT SIGNAL MANAGER (ISM)/SENSOR FUSION ==
  ACCL : Inport
  GYRO : Inport  Port=2
  MAG : Inport  Port=3
  " 1" : DataTypeConversion  OutDataTypeStr=double  SaturateOnIntegerOverflow=off  RndMeth=Floor
  " 2" : DataTypeConversion  OutDataTypeStr=double  SaturateOnIntegerOverflow=off  RndMeth=Floor
  "0 " : DataTypeConversion  OutDataTypeStr=double  SaturateOnIntegerOverflow=off  RndMeth=Floor
  AHRS : mspfiltlib/AHRS  DispRefFrame=NED  DecimationFactor=1  InitialProcessNoise=ahrsfilter.defaultProcessNoise  OrientationFormat=Rotation matrix  SimulateUsing=Interpreted execution  AccelerometerNoise=0.0001924722  GyroscopeNoise=9.1385e-5  MagnetometerNoise=0.1  GyroscopeDriftNoise=3.0462e-13  LinearAccelerationNoise=0.0096236100000000012  MagneticDisturbanceNoise=0.5  LinearAccelerationDecayFactor=0.5  MagneticDisturbanceDecayFactor=0.5  ExpectedMagneticFieldStrength=50
  SENSOR FUSION : Subsystem
  NED_ORIENTATION : Outport
  TRUE_ROLL : Outport  Port=2
  TRUE_PITCH : Outport  Port=3
  TRUE_YAW : Outport  Port=4
  wires:
  GYRO/1 -> AHRS/2
  ACCL/1 -> AHRS/1
  MAG/1 -> AHRS/3
  AHRS/1 -> NED_ORIENTATION/1
  AHRS/2 -> SENSOR FUSION/1(ANGULAR_VEL)
  SENSOR FUSION/1(TRUE_ROLL) -> "0 "/1
  SENSOR FUSION/2(TRUE_PITCH) -> " 1"/1
  SENSOR FUSION/3(TRUE_YAW) -> " 2"/1
  " 2"/1 -> TRUE_YAW/1
  " 1"/1 -> TRUE_PITCH/1
  "0 "/1 -> TRUE_ROLL/1

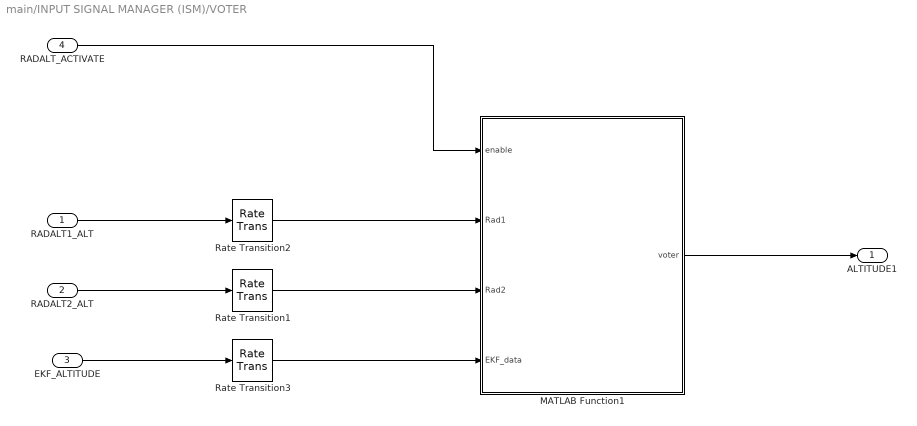
== system main/INPUT SIGNAL MANAGER (ISM)/VOTER ==
  RADALT1_ALT : Inport
  RADALT2_ALT : Inport  Port=2
  EKF_ALTITUDE : Inport  Port=3
  RADALT_ACTIVATE : Inport  Port=4
  MATLAB Function1 : MATLAB Function  TreatAsAtomicUnit=on
  Rate Transition1 : RateTransition
  Rate Transition2 : RateTransition
  Rate Transition3 : RateTransition
  ALTITUDE1 : Outport
  wires:
  RADALT_ACTIVATE/1 -> MATLAB Function1/1(enable)
  Rate Transition3/1 -> MATLAB Function1/4(EKF_data)
  Rate Transition1/1 -> MATLAB Function1/3(Rad2)
  MATLAB Function1/1(voter) -> ALTITUDE1/1
  EKF_ALTITUDE/1 -> Rate Transition3/1
  Rate Transition2/1 -> MATLAB Function1/2(Rad1)
  RADALT1_ALT/1 -> Rate Transition2/1
  RADALT2_ALT/1 -> Rate Transition1/1

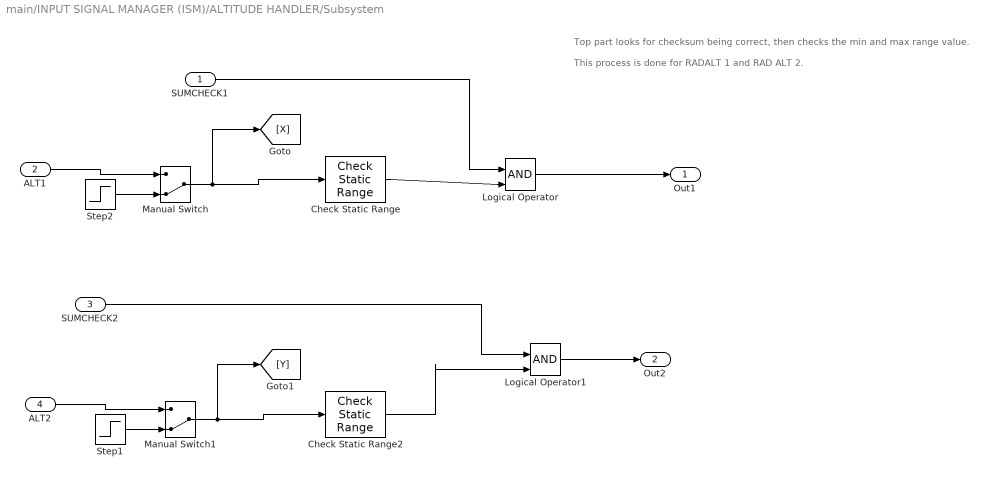
== system main/INPUT SIGNAL MANAGER (ISM)/ALTITUDE HANDLER/Subsystem ==
  note: This process is done for RADALT 1 and RAD ALT 2.
  note: Top part looks for checksum being correct, then checks the min and max range value.
  SUMCHECK1 : Inport
  ALT1 : Inport  Port=2
  SUMCHECK2 : Inport  Port=3
  ALT2 : Inport  Port=4
  Check Static Range : simulink/Model Verification/Check  Static Range  Description=Alt_min <= u <= Alt_max  max=Alt_max  max_included=on  min=Alt_min  min_included=on  enabled=on  stopWhenAssertionFail=off  export=on  icon=graphic
  Check Static Range2 : simulink/Model Verification/Check  Static Range  Description=Alt_min <= u <= Alt_max  max=Alt_max  max_included=on  min=Alt_min  min_included=on  enabled=on  stopWhenAssertionFail=off  export=on  icon=graphic
  Logical Operator : Logic  IconShape=distinctive  AllPortsSameDT=off  OutDataTypeStr=boolean
  Logical Operator1 : Logic  IconShape=distinctive  AllPortsSameDT=off  OutDataTypeStr=boolean
  Manual Switch : ManualSwitch  CurrentSetting=0
  Manual Switch1 : ManualSwitch  CurrentSetting=0
  Step1 : Step  Time=10  Before=5  After=0  SampleTime=10
  Step2 : Step  Time=10  Before=5  After=0  SampleTime=10
  Out1 : Outport
  Out2 : Outport  Port=2
  wires:
  Check Static Range/1 -> Logical Operator/2
  Logical Operator/1 -> Out1/1
  Check Static Range2/1 -> Logical Operator1/2
  Logical Operator1/1 -> Out2/1
  SUMCHECK1/1 -> Logical Operator/1
  SUMCHECK2/1 -> Logical Operator1/1
  Step2/1 -> Manual Switch/2
  ALT1/1 -> Manual Switch/1
  Manual Switch/1 -> [X], Check Static Range/1
  ALT2/1 -> Manual Switch1/1
  Step1/1 -> Manual Switch1/2
  Manual Switch1/1 -> [Y], Check Static Range2/1

== system main/INPUT SIGNAL MANAGER (ISM)/ALTITUDE HANDLER/Switch Case Action Subsystem ==
  ALT1 (cm) : Inport
  Action Port : ActionPort  ActionPortLabel=if(u1 == 1)
  Out1 : Outport
  wires:
  ALT1 (cm)/1 -> Out1/1

== system main/INPUT SIGNAL MANAGER (ISM)/ALTITUDE HANDLER/Switch Case Action Subsystem1 ==
  In1 : Inport
  Action Port : ActionPort  ActionPortLabel=else
  Out1 : Outport
  wires:
  In1/1 -> Out1/1

== system main/INPUT SIGNAL MANAGER (ISM)/ALTITUDE HANDLER/Switch Case Action Subsystem2 ==
  ALT2 (cm) : Inport
  Action Port : ActionPort  ActionPortLabel=if(u1 == 1)
  Out1 : Outport
  wires:
  ALT2 (cm)/1 -> Out1/1

== system main/INPUT SIGNAL MANAGER (ISM)/ALTITUDE HANDLER/Switch Case Action Subsystem3 ==
  In1 : Inport
  Action Port : ActionPort  ActionPortLabel=else
  Out1 : Outport
  wires:
  In1/1 -> Out1/1

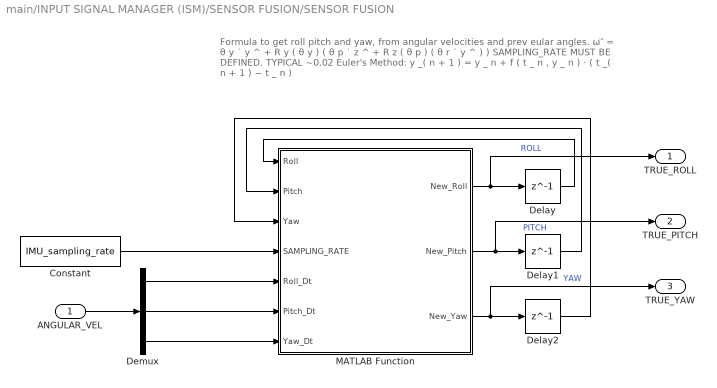
== system main/INPUT SIGNAL MANAGER (ISM)/SENSOR FUSION/SENSOR FUSION ==
  note: Formula to get roll pitch and yaw, from angular velocities and prev eular angles.
      | ω ⃗ = θ y ˙ y ^ + R y ( θ y ) ( θ p ˙ z ^ + R z ( θ p ) ( θ r ˙ y ^ ) )
      | SAMPLING_RATE MUST BE DEFINED. TYPICAL ~0.02
      | Euler's Method: y _( n + 1 ) = y _ n + f ( t _ n , y _ n ) ⋅ ( t _( n + 1 ) − t _ n )
  ANGULAR_VEL : Inport
  Constant : Constant  Value=IMU_sampling_rate
  Delay : Delay  DelayLength=1
  Delay1 : Delay  DelayLength=1
  Delay2 : Delay  DelayLength=1
  Demux : Demux  Outputs=3
  MATLAB Function : MATLAB Function  TreatAsAtomicUnit=on
  TRUE_ROLL : Outport
  TRUE_PITCH : Outport  Port=2
  TRUE_YAW : Outport  Port=3
  wires:
  MATLAB Function/1(New_Roll) -> TRUE_ROLL/1, Delay/1  "ROLL"
  Demux/2 -> MATLAB Function/6(Pitch_Dt)
  Delay1/1 -> MATLAB Function/2(Pitch)
  MATLAB Function/2(New_Pitch) -> TRUE_PITCH/1, Delay1/1  "PITCH"
  MATLAB Function/3(New_Yaw) -> TRUE_YAW/1, Delay2/1  "YAW"
  Delay/1 -> MATLAB Function/1(Roll)
  Delay2/1 -> MATLAB Function/3(Yaw)
  Demux/3 -> MATLAB Function/7(Yaw_Dt)
  Demux/1 -> MATLAB Function/5(Roll_Dt)
  ANGULAR_VEL/1 -> Demux/1
  Constant/1 -> MATLAB Function/4(SAMPLING_RATE)

== matlab function main/INPUT SIGNAL MANAGER (ISM)/VOTER/MATLAB Function1 ==
  data: enable input; Rad1 input; voter output; Rad2 input; EKF_data input
function voter = vote(enable,Rad1,Rad2,EKF_data)
EKF = EKF_data + 0.000000000001;
con1 = (Rad1 / EKF >= 0.85) && (Rad1 / EKF <= 1.15);
con2 = (Rad2 / EKF >= 0.85) && (Rad2 / EKF <= 1.15);
if enable == 0 
    voter = EKF_data;
    
elseif con1 && con2
    voter = (Rad1+Rad2)/2;
elseif con1 
    voter = (Rad1);
elseif con2
    voter = (Rad2);
else
    voter = EKF_data;
end

== matlab function main/INPUT SIGNAL MANAGER (ISM)/SENSOR FUSION/SENSOR FUSION/MATLAB Function ==
  data: Roll input; Pitch input; Yaw input; SAMPLING_RATE input; Roll_Dt input; Pitch_Dt input; Yaw_Dt input; New_Roll output; New_Pitch output; New_Yaw output
function [New_Roll,New_Pitch,New_Yaw] = EulerRatesToEulerAngles(Roll,Pitch,Yaw, SAMPLING_RATE, Roll_Dt,Pitch_Dt,Yaw_Dt)

    New_Roll    = (Roll_Dt * SAMPLING_RATE) + Roll;
    New_Pitch   = (Pitch_Dt * SAMPLING_RATE) + Pitch;
    New_Yaw     = (Yaw_Dt * SAMPLING_RATE) + Yaw;
end

== matlab function main/INPUT SIGNAL MANAGER (ISM)/EKF/MATLAB Function1 ==
  data: x_prev input; P_prev input; x_est output; z input; dt input; P_est output; R input
function [x_est, P_est] = kalmanFilterStep(x_prev, P_prev, z, dt, R)
    % kalmanFilterStep performs a single step of the Kalman filter.
    %
    % Inputs:
    %   x_prev - The previous state estimate (2x1 vector: [altitude; velocity])
    %   P_prev - The previous state covariance matrix (2x2 matrix)
    %   z      - The measurement vector (2x1 vector: [altitude_measurement; velocity_measurement])
    %   dt     - Time step (scalar)
    %   R      - Measurement noise covariance matrix (2x2 matrix)
    %
    % Outputs:
    %   x_est - Updated state estimate
    %   P_est - Updated state covariance matrix

    % Define the state transition matrix (F) for a constant velocity model
    F = [1 dt; 0 1];

    % Define the measurement matrix (H)
    H = [1 0; 0 1];
    
    % Assume no control input (B*u), but if there is, include it here
    % B = [...]; % Control input model
    % u = [...]; % Control input vector

    % Process noise covariance matrix (Q), assumed to be very small
    Q = [dt^2/4 dt/2; dt/2 dt] * 1e-4;

    % Prediction step
    x_pred = F * x_prev; % + B * u; (uncomment if control input is used)
    P_pred = F * P_prev * F' + Q;

    % Kalman Gain calculation
    K = P_pred * H' / (H * P_pred * H' + R);

    % Measurement Update step
    x_est = x_pred + K * (z - H * x_pred);
    P_est = (eye(2) - K * H) * P_pred;

end
